simulink model "DiscreteFilter2014b"  (Simulink 8.4)
settings: Solver=ode3  SolverMode=SingleTasking  StartTime=0.0  StopTime=10.0  FixedStep=0.01  RelTol=1e-3
libraries: WBToolboxLibrary x1
settings Model: Creator=icub  LastModifiedBy=icub  CovMetricSettings=dwe  CovHtmlReporting=off  covSaveCumulativeToWorkspaceVar=off  CovSaveSingleToWorkspaceVar=off  CovExternalEMLEnable=on  CovSFcnEnable=on
settings DataIOCC: LimitDataPoints=off  SaveFormat=StructureWithTime  SignalLoggingSaveFormat=Dataset
settings OptimizationCC: ExpressionDepthLimit=128
settings DebuggingCC: UnderspecifiedInitializationDetection=Simplified  MergeDetectMultiDrivingBlocksExec=error  SolverPrmCheckMsg=none  FcnCallInpInsideContextMsg=EnableAllAsError  FrameProcessingCompatibilityMsg=error  StateNameClashWarn=none  SFUnexpectedBacktrackingDiag=error  SFNoUnconditionalDefaultTransitionDiag=error
settings HardwareCC: ProdBitPerPointer=64  ProdLargestAtomicFloat=Float  ProdIntDivRoundTo=Zero  ProdEndianess=LittleEndian  ProdHWDeviceType=Specified
settings ModelReferenceCC: PropagateSignalLabelsOutOfModel=on
settings GRTTargetCC: TargetLangStandard=C99 (ISO)  GeneratePreprocessorConditionals=Use local settings  CombineOutputUpdateFcns=on  GRTInterface=off

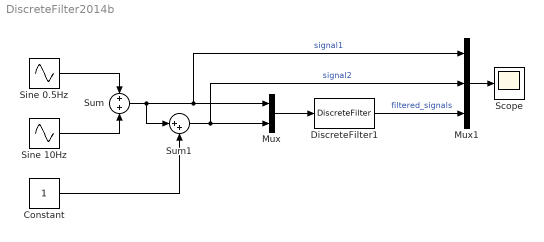
== system DiscreteFilter2014b ==
  Constant : Constant
  DiscreteFilter1 : WBToolboxLibrary/Utilities/DiscreteFilter  filterType=FirstOrderLowPassFilter  numCoeffs=[0]  denCoeffs=[0]  Fc=1  Ts=0.01  orderMedianFilter=0  initStatus=on  y0=[0 1]  u0=[0]
  Mux : Mux  Inputs=2
  Mux1 : Mux  Inputs=3
  Scope : Scope
      settings: TimeRange=auto  ShowLegends=on  MaxDataPoints=5000  SaveToWorkspace=off  SaveName=ScopeData  YMin=-1.6103  YMax=2.6103  SampleTime=-1
  Sine 0.5Hz : Sin  Frequency=2*pi*0.5  SampleTime=0
  Sine 10Hz : Sin  Amplitude=0.2  Frequency=2*pi*10  SampleTime=0
  Sum : Sum  Inputs=+|+
  Sum1 : Sum  Inputs=|++
  wires:
  DiscreteFilter1/1 -> Mux1/3  "filtered_signals"
  Sum/1 -> Mux1/1, Mux/1, Sum1/1  "signal1"
  Sine 0.5Hz/1 -> Sum/1
  Sine 10Hz/1 -> Sum/2
  Sum1/1 -> Mux1/2, Mux/2  "signal2"
  Constant/1 -> Sum1/2
  Mux/1 -> DiscreteFilter1/1
  Mux1/1 -> Scope/1
